simulink model "assignmentEE"  (R2021b)
settings: Solver=VariableStepAuto  StartTime=0.0  StopTime=10.0  MaxStep=0.02  RelTol=1e-3
settings Model: Creator=emil1  LastModifiedBy=emil1

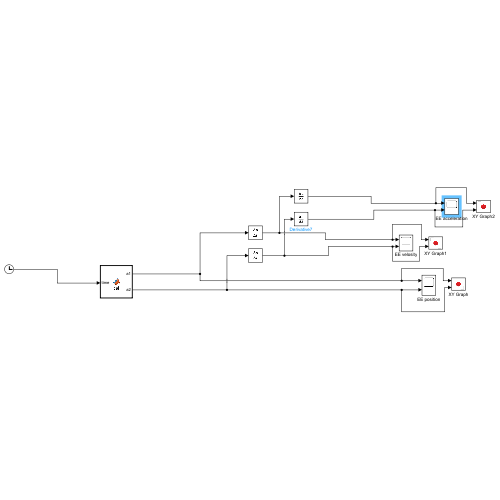
[thumbnail: Simulink's stored preview of the top-level diagram]
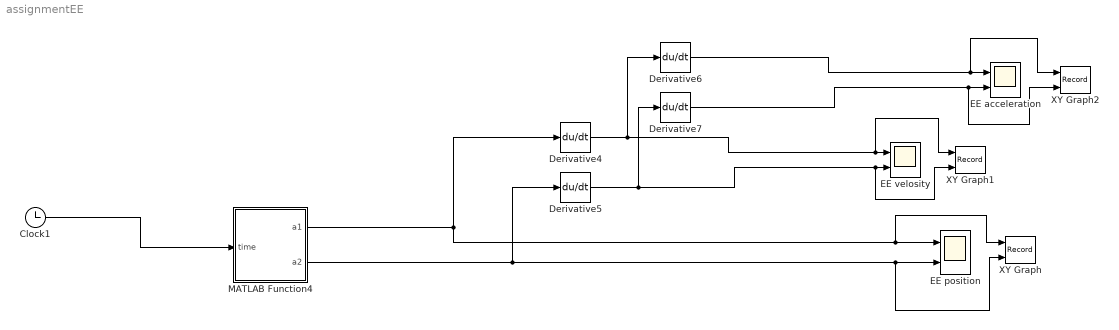
== system assignmentEE ==
  Clock1 : Clock
  Derivative{4..7} (4 alike) : Derivative
  EE acceleration : Scope  NumInputPorts=2
  EE position : Scope  NumInputPorts=2
  EE velosity : Scope  NumInputPorts=2
  MATLAB Function4 : MATLAB Function  TreatAsAtomicUnit=on
  XY Graph : Record  FileSettingsInternal="{\"entries\":[{\"content\":{\"excelSettings\":{\"content\":{},\"type\":\"Streamout.ExcelSettings\"}},\"type\":\"Streamout.FileSettingStorage\",\"uuid\":\"64e0a967-8a83-45eb-b41d-3a0058831dcc\"}],\"packageUris\":[\"http://schema.mathworks.com/mf0/streamout_blocks/R2020a\"],\"version\":\"1.0\"}"  Layout=[1 1]  SignalsInternal="{\"entries\":[{\"content\":{\"signals\":[{\"content\":{\"blockPath\":[\"untitled1/XY Graph\"],\"channel\":[],\"dimensions\":[1],\"domain\":\"untitled1/XY Graph\",\"lineColor\":\"#a2142f\",\"plots\":[1],\"port\":1,\"sid\":[\"\"],\"signalID\":1157,\"signalName\":\"MATLAB Function4:1\"},\"type\":\"RecordBlkView.Signal\",\"uuid\":\"91f3641e-e947-424d-ae64-3bec539cc820\"},{\"content\":{\"blockPath\":[\"untitled1/XY Graph\"],\"channel\":[],\"dimensions\":[1],\"domain\":\"untitled1/XY Graph\",\"lineColor\":\"#139fff\",\"plots\":[1],\"port\":2,\"sid\":[\"\"],\"signalID\":1161,\"signalName\":\"MATLAB Function4:2\"},\"type\":\"RecordBlkView.Signal\",\"uuid\":\"2a23e264-2b79-4ff5-b853-282124cd4e19\"}]},\"type\":\"RecordBlkView.InputSignals\",\"uuid\":\"d6161ed4-66ec-4442-91ca-7fd72cef1b6e\"}],\"packageUris\":[\"http://schema.mathworks.com/mf0/streamout_blocks/R2020a\"],\"version\":\"1.0\"}"  VisualizationBindings="{\"xyplotplugin\":{\"info\":[{\"series\":[{\"bindingParametersList\":[{\"parameter\":\"X-Axis\",\"signalID\":1157,\"signalName\":\"MATLAB Function4:1\"},{\"parameter\":\"Y-Axis\",\"signalID\":1161,\"signalName\":\"MATLAB Function4:2\"}],\"seriesID\":20837}],\"subplotID\":1}]}}"  CompatibilityTag=XY
  XY Graph1 : Record  FileSettingsInternal="{\"entries\":[{\"content\":{\"excelSettings\":{\"content\":{},\"type\":\"Streamout.ExcelSettings\"}},\"type\":\"Streamout.FileSettingStorage\",\"uuid\":\"e42d7738-f59f-421f-8156-738de62e0d3f\"}],\"packageUris\":[\"http://schema.mathworks.com/mf0/streamout_blocks/R2020a\"],\"version\":\"1.0\"}"  Layout=[1 1]  SignalsInternal="{\"entries\":[{\"content\":{\"signals\":[{\"content\":{\"blockPath\":[\"untitled1/XY Graph1\"],\"channel\":[],\"dimensions\":[1],\"domain\":\"untitled1/XY Graph1\",\"lineColor\":\"#a2142f\",\"plots\":[1],\"port\":1,\"sid\":[\"\"],\"signalID\":1165,\"signalName\":\"Derivative4\"},\"type\":\"RecordBlkView.Signal\",\"uuid\":\"313c79c5-d2cf-4ecf-8e0c-94e512aab61e\"},{\"content\":{\"blockPath\":[\"untitled1/XY Graph1\"],\"channel\":[],\"dimensions\":[1],\"domain\":\"untitled1/XY Graph1\",\"lineColor\":\"#139fff\",\"plots\":[1],\"port\":2,\"sid\":[\"\"],\"signalID\":1169,\"signalName\":\"Derivative5\"},\"type\":\"RecordBlkView.Signal\",\"uuid\":\"623a07c8-7d05-4183-98f5-0258c0034a02\"}]},\"type\":\"RecordBlkView.InputSignals\",\"uuid\":\"83e98cef-799c-45f2-9db1-38dce95d23b5\"}],\"packageUris\":[\"http://schema.mathworks.com/mf0/streamout_blocks/R2020a\"],\"version\":\"1.0\"}"  VisualizationBindings="{\"xyplotplugin\":{\"info\":[{\"series\":[{\"bindingParametersList\":[{\"parameter\":\"X-Axis\",\"signalID\":1165,\"signalName\":\"Derivative4\"},{\"parameter\":\"Y-Axis\",\"signalID\":1169,\"signalName\":\"Derivative5\"}],\"seriesID\":36194}],\"subplotID\":1}]}}"  CompatibilityTag=XY
  XY Graph2 : Record  FileSettingsInternal="{\"entries\":[{\"content\":{\"excelSettings\":{\"content\":{},\"type\":\"Streamout.ExcelSettings\"}},\"type\":\"Streamout.FileSettingStorage\",\"uuid\":\"d81d0d79-89e9-44cb-95cf-999b9d242173\"}],\"packageUris\":[\"http://schema.mathworks.com/mf0/streamout_blocks/R2020a\"],\"version\":\"1.0\"}"  Layout=[1 1]  SignalsInternal="{\"entries\":[{\"content\":{\"signals\":[{\"content\":{\"blockPath\":[\"untitled1/XY Graph2\"],\"channel\":[],\"dimensions\":[1],\"domain\":\"untitled1/XY Graph2\",\"lineColor\":\"#a2142f\",\"plots\":[1],\"port\":1,\"sid\":[\"\"],\"signalID\":1173,\"signalName\":\"Derivative6\"},\"type\":\"RecordBlkView.Signal\",\"uuid\":\"d3be1499-ddbb-4d15-bea9-be450a8addee\"},{\"content\":{\"blockPath\":[\"untitled1/XY Graph2\"],\"channel\":[],\"dimensions\":[1],\"domain\":\"untitled1/XY Graph2\",\"lineColor\":\"#139fff\",\"plots\":[1],\"port\":2,\"sid\":[\"\"],\"signalID\":1177,\"signalName\":\"Derivative7\"},\"type\":\"RecordBlkView.Signal\",\"uuid\":\"b4f8bbfb-192b-4c8d-97dd-1bc90dc90e3a\"}]},\"type\":\"RecordBlkView.InputSignals\",\"uuid\":\"6f071c64-6230-496a-a1d5-c8b43dedfb66\"}],\"packageUris\":[\"http://schema.mathworks.com/mf0/streamout_blocks/R2020a\"],\"version\":\"1.0\"}"  VisualizationBindings="{\"xyplotplugin\":{\"info\":[{\"series\":[{\"bindingParametersList\":[{\"parameter\":\"X-Axis\",\"signalID\":1173,\"signalName\":\"Derivative6\"},{\"parameter\":\"Y-Axis\",\"signalID\":1177,\"signalName\":\"Derivative7\"}],\"seriesID\":57217}],\"subplotID\":1}]}}"  CompatibilityTag=XY
  wires:
  MATLAB Function4/2(a2) -> Derivative5/1, EE position/2, XY Graph/2
  Clock1/1 -> MATLAB Function4/1(time)
  Derivative5/1 -> Derivative7/1, XY Graph1/2, EE velosity/2
  MATLAB Function4/1(a1) -> XY Graph/1, EE position/1, Derivative4/1
  Derivative4/1 -> Derivative6/1, XY Graph1/1, EE velosity/1
  Derivative6/1 -> EE acceleration/1, XY Graph2/1
  Derivative7/1 -> EE acceleration/2, XY Graph2/2

== matlab function assignmentEE/MATLAB Function4 ==
  data: time input; a1 output; a2 output
function [a1, a2]= cal(time)
 

radian = pi*45/180;

theta_1 = 3*sin(pi*time);

theta_2 = 0.5*sin(pi*3*time + radian);

l1 = 1;

l2 = 0.5;

a = [l2*cos(theta_1+theta_2)+l1*cos(theta_1) l2*sin(theta_2+theta_1)+l1*sin(theta_1)];


a1=a(1);

a2=a(2);
